simulink model "Ex3"  (R2019a)
settings: Solver=VariableStepAuto  StartTime=0.0  StopTime=10.0  RelTol=1e-3
settings Model: Creator=G5  LastModifiedBy=G5

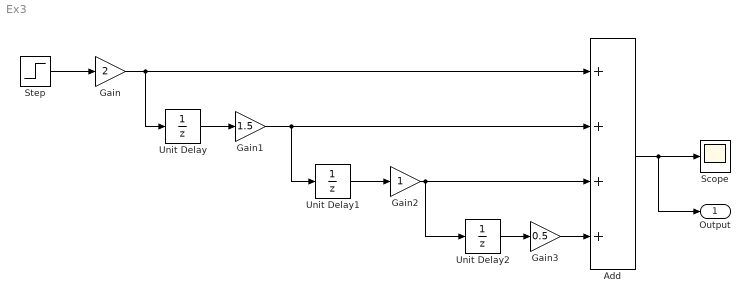
== system Ex3 ==
  Add : Sum  Inputs=++++
  Gain : Gain  Gain=2  SampleTime=20
  Gain1 : Gain  Gain=1.5  SampleTime=20
  Gain2 : Gain  SampleTime=20
  Gain3 : Gain  Gain=0.5  SampleTime=20
  Scope : Scope
  Step : Step  SampleTime=0
  Unit Delay : UnitDelay  SampleTime=-1  HasFrameUpgradeWarning=on
  Unit Delay1 : UnitDelay  SampleTime=-1  HasFrameUpgradeWarning=on
  Unit Delay2 : UnitDelay  SampleTime=-1  HasFrameUpgradeWarning=on
  Output : Outport
  wires:
  Step/1 -> Gain/1
  Gain/1 -> Add/1, Unit Delay/1
  Unit Delay/1 -> Gain1/1
  Gain1/1 -> Add/2, Unit Delay1/1
  Unit Delay1/1 -> Gain2/1
  Gain2/1 -> Unit Delay2/1, Add/3
  Unit Delay2/1 -> Gain3/1
  Gain3/1 -> Add/4
  Add/1 -> Output/1, Scope/1
